simulink model "Ripple_factor_rectifier_single_phase"  (R2024b)
settings: Solver=ode3  StartTime=0.0  StopTime=4/50  FixedStep=10e-6  RelTol=1e-3
libraries: spsDiodeLib x5, spsSeriesRLCBranchLib x4, spsVoltageMeasurementLib x4, spsACVoltageSourceLib x2, sps_lib x1
settings Model: Creator=Abhijith_Kumble  LastModifiedBy=Abhijith_Kumble

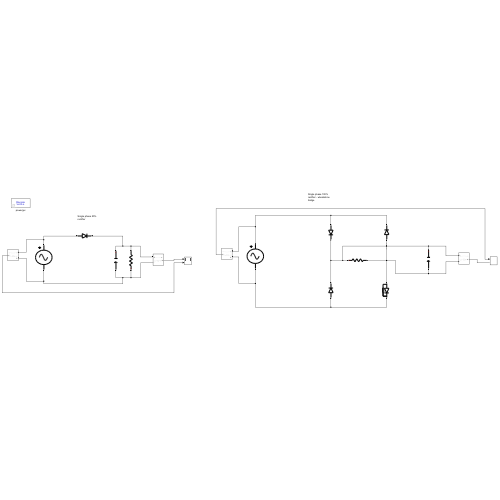
[thumbnail: Simulink's stored preview of the top-level diagram]
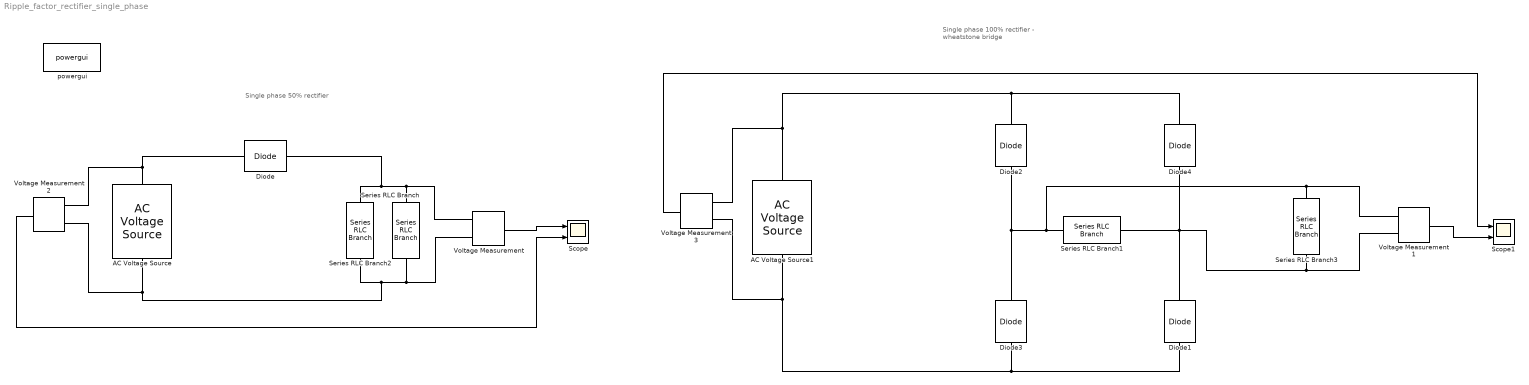
== system Ripple_factor_rectifier_single_phase ==
  note: Single phase 50% rectifier
  note: Single phase 100% rectifier - wheatstone bridge
  AC Voltage Source : spsACVoltageSourceLib/AC Voltage Source  Amplitude=230  Phase=0  Frequency=50  SampleTime=0  Measurements=None  BusType=swing  Pref=10e3  Qref=0  Qmin=-inf  Qmax=+inf
  AC Voltage Source1 : spsACVoltageSourceLib/AC Voltage Source  Amplitude=230  Phase=0  Frequency=50  SampleTime=0  Measurements=None  BusType=swing  Pref=10e3  Qref=0  Qmin=-inf  Qmax=+inf
  Diode : spsDiodeLib/Diode  Ron=0.001  Lon=0  Vf=0.0  IC=0  UseSnubber=0  Rs=0  Cs=0  Measurements=off
  Diode1 : spsDiodeLib/Diode  Ron=0.001  Lon=0  Vf=0.8  IC=0  UseSnubber=0  Rs=0  Cs=1e-6  Measurements=off
  Diode2 : spsDiodeLib/Diode  Ron=0.001  Lon=0  Vf=0.8  IC=0  UseSnubber=0  Rs=0  Cs=0  Measurements=off
  Diode3 : spsDiodeLib/Diode  Ron=0.001  Lon=0  Vf=0.8  IC=0  UseSnubber=0  Rs=0  Cs=0  Measurements=off
  Diode4 : spsDiodeLib/Diode  Ron=0.001  Lon=0  Vf=0.8  IC=0  UseSnubber=0  Rs=0  Cs=0  Measurements=off
  Scope : Scope  NumInputPorts=2
  Scope1 : Scope  NumInputPorts=2
  Series RLC Branch : spsSeriesRLCBranchLib/Series RLC Branch  LConnTagsString=__new0  RConnTagsString=__new0  BranchType=R  Resistance=1000  Inductance=1e-3  SetiL0=off  InitialCurrent=0  Capacitance=1e-6  Setx0=off  InitialVoltage=0  Measurements=None
  Series RLC Branch1 : spsSeriesRLCBranchLib/Series RLC Branch  LConnTagsString=__new0  RConnTagsString=__new0  BranchType=R  Resistance=1000  Inductance=1e-3  SetiL0=off  InitialCurrent=0  Capacitance=1e-6  Setx0=off  InitialVoltage=0  Measurements=None
  Series RLC Branch2 : spsSeriesRLCBranchLib/Series RLC Branch  LConnTagsString=__new0  RConnTagsString=__new0  BranchType=C  Resistance=1  Inductance=1e-3  SetiL0=off  InitialCurrent=0  Capacitance=20*10e-6  Setx0=off  InitialVoltage=0  Measurements=None
  Series RLC Branch3 : spsSeriesRLCBranchLib/Series RLC Branch  LConnTagsString=__new0  RConnTagsString=__new0  BranchType=C  Resistance=1  Inductance=1e-3  SetiL0=off  InitialCurrent=0  Capacitance=100e-6  Setx0=off  InitialVoltage=0  Measurements=None
  Voltage Measurement{,1..3} (4 alike) : spsVoltageMeasurementLib/Voltage Measurement  PhasorSimulation=off  OutputType=Complex  PSBequivalent=0
  powergui : sps_lib/powergui  Priority=1  SimulationMode=Discrete  SampleTime=10e-6  frequency=50  Iterations=50  frequencyindice=50  Pbase=100e6  ErrMax=1e-4  UnitsV=kV  UnitsW=MW  buscounter=0  FunctionMessages=off  echomessages=off  EnableUseOfTLC=off  CurrentSourceSwitches=off  DisableSnubberDevices=off  DisableRonSwitches=off  DisableVfSwitches=off  DisplayEquations=off  AutomaticDiscreteSolvers=off  SolverType=Tustin/Backward Euler (TBE)  Interpol=off  ExternalGateDelay=off  methode=off  Ts=100  x0status=blocks  SPID=on  SwTol=0  HookPort=off  NonlinearTolerance=1e-4  nMaxIteration=100  ContinueOnMaxIteration=off  RestoreLinks=warning  ResistiveCurrentMeasurement=off  Frange=[0:2:500]  Ylog=off  Xlog=on  ShowGrid=off  save=off  variable=ZData  structure=0  ZoomFFT=off  StartTime=0.0  cycles=1  DisplayStyle=1  fundamental=60  FreqAxis=off  MaxFrequency=1000  frequencyindicesteady=1  RmsSteady=1  display=off
  wires:
  Voltage Measurement/1 -> Scope/1
  Voltage Measurement1/1 -> Scope1/2
  Voltage Measurement2/1 -> Scope/2
  Voltage Measurement3/1 -> Scope1/1
  connections:
  Diode/LConn1 -- Voltage Measurement2/LConn2 -- AC Voltage Source/RConn1
  AC Voltage Source/LConn1 -- Voltage Measurement2/LConn1 -- Voltage Measurement/LConn2 -- Series RLC Branch/LConn1 -- Series RLC Branch2/RConn1
  Series RLC Branch/RConn1 -- Series RLC Branch2/LConn1 -- Diode/RConn1 -- Voltage Measurement/LConn1
  Diode4/RConn1 -- AC Voltage Source1/RConn1 -- Voltage Measurement3/LConn2 -- Diode2/LConn1
  AC Voltage Source1/LConn1 -- Voltage Measurement3/LConn1 -- Diode1/RConn1 -- Diode3/LConn1
  Series RLC Branch1/LConn1 -- Series RLC Branch3/LConn1 -- Voltage Measurement1/LConn1 -- Diode2/RConn1 -- Diode3/RConn1
  Series RLC Branch1/RConn1 -- Diode4/LConn1 -- Diode1/LConn1 -- Series RLC Branch3/RConn1 -- Voltage Measurement1/LConn2
